simulink model "unrolling_1"  (R2015b)
settings: Solver=FixedStepDiscrete  SolverMode=SingleTasking  StartTime=0.0  StopTime=10.0  RelTol=1e-3
undefined symbols (not defined in the file or in its folder): a, b
libraries: shlslibv1 x4645
(part 1 of 18)
settings Model: synDspstartup=OK  Creator=hchempat  LastModifiedBy=pjampani
settings DataIOCC: SaveOutput=off  SignalLogging=off  SaveTime=off
settings OptimizationCC: DefaultParameterBehavior=Inlined
settings DebuggingCC: AlgebraicLoopMsg=error  InheritedTsInSrcMsg=none

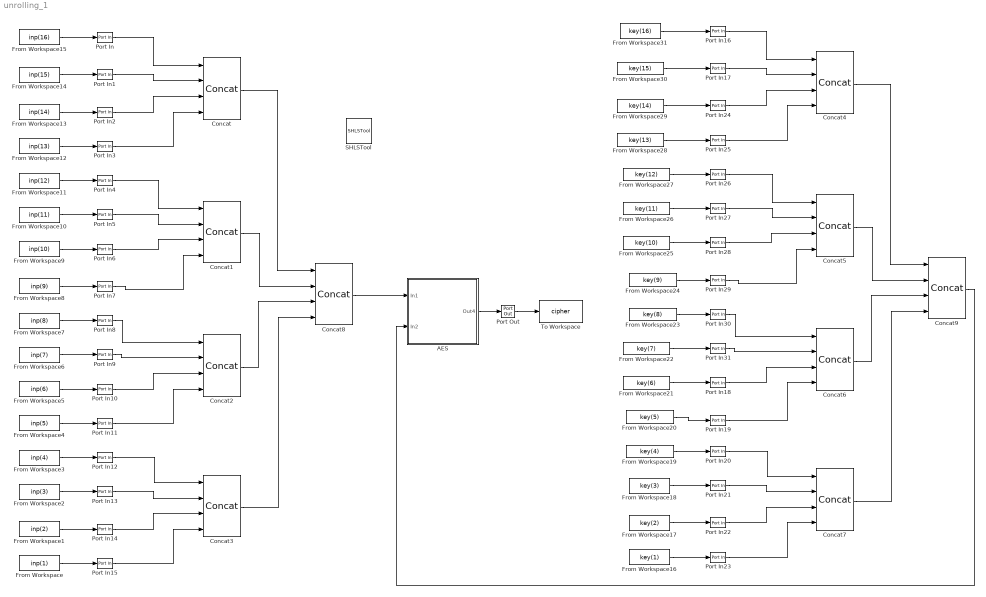
== system unrolling_1 ==
  "AES " : Subsystem
  Concat{,1..9} (10 alike) : shlslibv1/Signal Operations/Concat  syn_in_nb=4  syn_out_f=Automatic  syn_out_wl=16  syn_out_fl=8  syn_out_dt=signed  syn_en_se=off  synBlockType=primitive  synLatency=0  synBlockId=8
  From Workspace : FromWorkspace  VariableName=inp(1)
  From Workspace1 : FromWorkspace  VariableName=inp(2)
  From Workspace10 : FromWorkspace  VariableName=inp(11)
  From Workspace11 : FromWorkspace  VariableName=inp(12)
  From Workspace12 : FromWorkspace  VariableName=inp(13)
  From Workspace13 : FromWorkspace  VariableName=inp(14)
  From Workspace14 : FromWorkspace  VariableName=inp(15)
  From Workspace15 : FromWorkspace  VariableName=inp(16)
  From Workspace16 : FromWorkspace  VariableName=key(1)
  From Workspace17 : FromWorkspace  VariableName=key(2)
  From Workspace18 : FromWorkspace  VariableName=key(3)
  From Workspace19 : FromWorkspace  VariableName=key(4)
  From Workspace2 : FromWorkspace  VariableName=inp(3)
  From Workspace20 : FromWorkspace  VariableName=key(5)
  From Workspace21 : FromWorkspace  VariableName=key(6)
  From Workspace22 : FromWorkspace  VariableName=key(7)
  From Workspace23 : FromWorkspace  VariableName=key(8)
  From Workspace24 : FromWorkspace  VariableName=key(9)
  From Workspace25 : FromWorkspace  VariableName=key(10)
  From Workspace26 : FromWorkspace  VariableName=key(11)
  From Workspace27 : FromWorkspace  VariableName=key(12)
  From Workspace28 : FromWorkspace  VariableName=key(13)
  From Workspace29 : FromWorkspace  VariableName=key(14)
  From Workspace3 : FromWorkspace  VariableName=inp(4)
  From Workspace30 : FromWorkspace  VariableName=key(15)
  From Workspace31 : FromWorkspace  VariableName=key(16)
  From Workspace4 : FromWorkspace  VariableName=inp(5)
  From Workspace5 : FromWorkspace  VariableName=inp(6)
  From Workspace6 : FromWorkspace  VariableName=inp(7)
  From Workspace7 : FromWorkspace  VariableName=inp(8)
  From Workspace8 : FromWorkspace  VariableName=inp(9)
  From Workspace9 : FromWorkspace  VariableName=inp(10)
  Port In{,1..31} (32 alike) : shlslibv1/Ports & Subsystems/Port In  syn_out_wl=8  syn_out_fl=0  syn_out_dt=unsigned  syn_out_st=ts  syn_capture=on  syn_register=on  syn_out_sat=off  syn_out_rnd=on  synBlockType=port  synLatency=1  synBlockId=0
  Port Out : shlslibv1/Ports & Subsystems/Port Out  syn_capture=on  syn_register=on  synBlockType=port  synLatency=1  synBlockId=1
  SHLSTool : shlslibv1/SHLSTool  synBlockType=tool  syn_dsp_mode=FPGA
  To Workspace : ToWorkspace  VariableName=cipher  SaveFormat=Structure With Time  SampleTime=-1
  wires:
  From Workspace15/1 -> Port In/1
  From Workspace14/1 -> Port In1/1
  From Workspace12/1 -> Port In3/1
  From Workspace13/1 -> Port In2/1
  From Workspace11/1 -> Port In4/1
  From Workspace10/1 -> Port In5/1
  From Workspace9/1 -> Port In6/1
  From Workspace8/1 -> Port In7/1
  From Workspace7/1 -> Port In8/1
  From Workspace6/1 -> Port In9/1
  From Workspace5/1 -> Port In10/1
  From Workspace4/1 -> Port In11/1
  From Workspace3/1 -> Port In12/1
  From Workspace2/1 -> Port In13/1
  From Workspace1/1 -> Port In14/1
  From Workspace/1 -> Port In15/1
  Port In2/1 -> Concat/3
  Port In1/1 -> Concat/2
  Port In/1 -> Concat/1
  Port In3/1 -> Concat/4
  Port In6/1 -> Concat1/3
  Port In5/1 -> Concat1/2
  Port In4/1 -> Concat1/1
  Port In7/1 -> Concat1/4
  Port In10/1 -> Concat2/3
  Port In9/1 -> Concat2/2
  Port In8/1 -> Concat2/1
  Port In11/1 -> Concat2/4
  Port In14/1 -> Concat3/3
  Port In13/1 -> Concat3/2
  Port In15/1 -> Concat3/4
  Port In12/1 -> Concat3/1
  From Workspace22/1 -> Port In31/1
  From Workspace21/1 -> Port In18/1
  From Workspace20/1 -> Port In19/1
  From Workspace18/1 -> Port In21/1
  From Workspace17/1 -> Port In22/1
  From Workspace16/1 -> Port In23/1
  Port In24/1 -> Concat4/3
  Port In17/1 -> Concat4/2
  Port In16/1 -> Concat4/1
  Port In25/1 -> Concat4/4
  Port In28/1 -> Concat5/3
  Port In27/1 -> Concat5/2
  Port In26/1 -> Concat5/1
  Port In29/1 -> Concat5/4
  Port In18/1 -> Concat6/3
  Port In31/1 -> Concat6/2
  Port In30/1 -> Concat6/1
  Port In19/1 -> Concat6/4
  Port In22/1 -> Concat7/3
  Port In21/1 -> Concat7/2
  Port In23/1 -> Concat7/4
  Port In20/1 -> Concat7/1
  Concat/1 -> Concat8/1
  Concat1/1 -> Concat8/2
  Concat2/1 -> Concat8/3
  Concat3/1 -> Concat8/4
  Concat4/1 -> Concat9/1
  Concat5/1 -> Concat9/2
  Concat6/1 -> Concat9/3
  Concat7/1 -> Concat9/4
  Port Out/1 -> To Workspace/1
  Concat8/1 -> "AES "/1(In1)
  Concat9/1 -> "AES "/2(In2)
  "AES "/1(Out4) -> Port Out/1
  From Workspace19/1 -> Port In20/1
  From Workspace23/1 -> Port In30/1
  From Workspace24/1 -> Port In29/1
  From Workspace25/1 -> Port In28/1
  From Workspace27/1 -> Port In26/1
  From Workspace28/1 -> Port In25/1
  From Workspace29/1 -> Port In24/1
  From Workspace30/1 -> Port In17/1
  From Workspace31/1 -> Port In16/1
  From Workspace26/1 -> Port In27/1

== system unrolling_1/AES  ==
  In1 : Inport
  In2 : Inport  Port=2
  Concat : shlslibv1/Signal Operations/Concat  syn_in_nb=4  syn_out_f=Automatic  syn_out_wl=16  syn_out_fl=8  syn_out_dt=signed  syn_en_se=off  synBlockType=primitive  synLatency=0  synBlockId=8
  Subsystem : Subsystem
  Subsystem1 : Subsystem
  Subsystem10 : Subsystem
  Subsystem2 : Subsystem
  Subsystem3 : Subsystem
  Subsystem4 : Subsystem
  Subsystem5 : Subsystem
  Subsystem6 : Subsystem
  Subsystem7 : Subsystem
  Subsystem8 : Subsystem
  Subsystem9 : Subsystem
  Out4 : Outport
  wires:
  Subsystem/1(Out1) -> Subsystem1/1(In1)
  Subsystem/2(Out2) -> Subsystem1/2(In2)
  Subsystem/3(Out3) -> Subsystem1/3(In3)
  Subsystem/4(Out4) -> Subsystem1/4(In4)
  Subsystem1/1(Out1) -> Subsystem2/1(In1)
  Subsystem1/2(Out2) -> Subsystem2/2(In2)
  Subsystem1/3(Out3) -> Subsystem2/3(In3)
  Subsystem1/4(Out4) -> Subsystem2/4(In4)
  Subsystem1/5(Out5) -> Subsystem2/5(In5)
  Subsystem2/1(Out1) -> Subsystem3/1(In1)
  Subsystem2/2(Out2) -> Subsystem3/2(In2)
  Subsystem2/3(Out3) -> Subsystem3/3(In3)
  Subsystem2/4(Out4) -> Subsystem3/4(In4)
  Subsystem2/5(Out5) -> Subsystem3/5(In5)
  Subsystem3/1(Out1) -> Subsystem4/1(In1)
  Subsystem3/2(Out2) -> Subsystem4/2(In2)
  Subsystem3/3(Out3) -> Subsystem4/3(In3)
  Subsystem3/4(Out4) -> Subsystem4/4(In4)
  Subsystem3/5(Out5) -> Subsystem4/5(In5)
  Subsystem4/1(Out1) -> Subsystem5/1(In1)
  Subsystem4/2(Out2) -> Subsystem5/2(In2)
  Subsystem4/3(Out3) -> Subsystem5/3(In3)
  Subsystem4/4(Out4) -> Subsystem5/4(In4)
  Subsystem4/5(Out5) -> Subsystem5/5(In5)
  Subsystem5/1(Out1) -> Subsystem6/1(In1)
  Subsystem5/2(Out2) -> Subsystem6/2(In2)
  Subsystem5/3(Out3) -> Subsystem6/3(In3)
  Subsystem5/4(Out4) -> Subsystem6/4(In4)
  Subsystem5/5(Out5) -> Subsystem6/5(In5)
  Subsystem6/1(Out1) -> Subsystem7/1(In1)
  Subsystem6/2(Out2) -> Subsystem7/2(In2)
  Subsystem6/3(Out3) -> Subsystem7/3(In3)
  Subsystem6/4(Out4) -> Subsystem7/4(In4)
  Subsystem6/5(Out5) -> Subsystem7/5(In5)
  Subsystem7/5(Out5) -> Subsystem8/5(In5)
  Subsystem7/4(Out4) -> Subsystem8/4(In4)
  Subsystem7/3(Out3) -> Subsystem8/3(In3)
  Subsystem7/2(Out2) -> Subsystem8/2(In2)
  Subsystem8/1(Out1) -> Subsystem9/1(In1)
  Subsystem8/2(Out2) -> Subsystem9/2(In2)
  Subsystem8/5(Out5) -> Subsystem9/5(In5)
  Subsystem8/4(Out4) -> Subsystem9/4(In4)
  Subsystem8/3(Out3) -> Subsystem9/3(In3)
  Subsystem9/1(Out1) -> Subsystem10/1(In1)
  Subsystem9/2(Out2) -> Subsystem10/2(In2)
  Subsystem9/3(Out3) -> Subsystem10/3(In3)
  Subsystem9/4(Out4) -> Subsystem10/4(In4)
  Subsystem9/5(Out5) -> Subsystem10/5(In5)
  Subsystem10/4(Out4) -> Concat/4
  Subsystem10/3(Out3) -> Concat/3
  Subsystem10/2(Out2) -> Concat/2
  Subsystem10/1(Out1) -> Concat/1
  In2/1 -> Subsystem1/5(In5), Subsystem/2(In2)
  In1/1 -> Subsystem/1(In1)
  Concat/1 -> Out4/1
  Subsystem7/1(Out1) -> Subsystem8/1(In1)

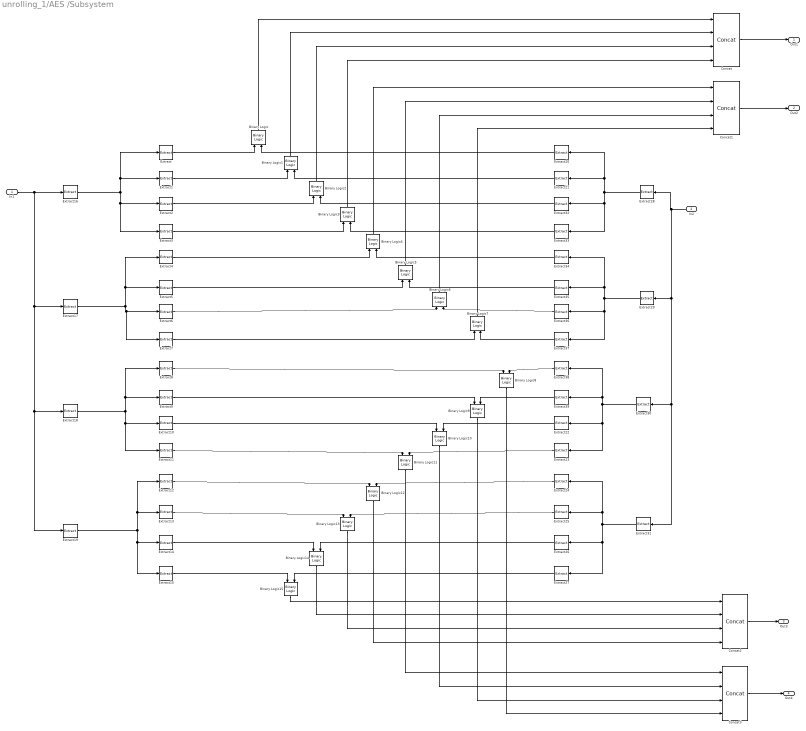
== system unrolling_1/AES /Subsystem ==
  In1 : Inport
  In2 : Inport  Port=2
  Binary Logic{,1..15} (16 alike) : shlslibv1/Math Functions/Binary Logic  syn_binlog_exp=a^b  synBlockType=primitive  synLatency=0  synBlockId=13
  Concat{,1..3} (4 alike) : shlslibv1/Signal Operations/Concat  syn_in_nb=4  syn_out_f=Automatic  syn_out_wl=16  syn_out_fl=8  syn_out_dt=signed  syn_en_se=off  synBlockType=primitive  synLatency=0  synBlockId=8
  Extract{,4,8,12,20,24,34,38} (8 alike) : shlslibv1/Signal Operations/Extract  syn_extract_vec=[24:31]  synBlockType=primitive  synLatency=0  synBlockId=17
  Extract{1,5,9,13,21,25,35,39} (8 alike) : shlslibv1/Signal Operations/Extract  syn_extract_vec=[16:23]  synBlockType=primitive  synLatency=0  synBlockId=17
  Extract{2,6,10,14,22,26,32,36} (8 alike) : shlslibv1/Signal Operations/Extract  syn_extract_vec=[8:15]  synBlockType=primitive  synLatency=0  synBlockId=17
  Extract{3,7,11,15,23,27,33,37} (8 alike) : shlslibv1/Signal Operations/Extract  syn_extract_vec=[0:7]  synBlockType=primitive  synLatency=0  synBlockId=17
  Extract16 : shlslibv1/Signal Operations/Extract  syn_extract_vec=[96:127]  synBlockType=primitive  synLatency=0  synBlockId=17
  Extract17 : shlslibv1/Signal Operations/Extract  syn_extract_vec=[64:95]  synBlockType=primitive  synLatency=0  synBlockId=17
  Extract18 : shlslibv1/Signal Operations/Extract  syn_extract_vec=[32:63]  synBlockType=primitive  synLatency=0  synBlockId=17
  Extract19 : shlslibv1/Signal Operations/Extract  syn_extract_vec=[0:31]  synBlockType=primitive  synLatency=0  synBlockId=17
  Extract28 : shlslibv1/Signal Operations/Extract  syn_extract_vec=[96:127]  synBlockType=primitive  synLatency=0  synBlockId=17
  Extract29 : shlslibv1/Signal Operations/Extract  syn_extract_vec=[64:95]  synBlockType=primitive  synLatency=0  synBlockId=17
  Extract30 : shlslibv1/Signal Operations/Extract  syn_extract_vec=[32:63]  synBlockType=primitive  synLatency=0  synBlockId=17
  Extract31 : shlslibv1/Signal Operations/Extract  syn_extract_vec=[0:31]  synBlockType=primitive  synLatency=0  synBlockId=17
  Out1 : Outport
  Out2 : Outport  Port=2
  Out3 : Outport  Port=3
  Out4 : Outport  Port=4
  wires:
  Extract16/1 -> Extract/1, Extract1/1, Extract2/1, Extract3/1
  Extract17/1 -> Extract6/1, Extract7/1, Extract4/1, Extract5/1
  Extract18/1 -> Extract9/1, Extract8/1, Extract10/1, Extract11/1
  Extract19/1 -> Extract12/1, Extract13/1, Extract15/1, Extract14/1
  In1/1 -> Extract19/1, Extract18/1, Extract17/1, Extract16/1
  In2/1 -> Extract31/1, Extract30/1, Extract29/1, Extract28/1
  Extract28/1 -> Extract21/1, Extract20/1, Extract33/1, Extract32/1
  Extract29/1 -> Extract35/1, Extract34/1, Extract36/1, Extract37/1
  Extract30/1 -> Extract23/1, Extract22/1, Extract38/1, Extract39/1
  Extract31/1 -> Extract24/1, Extract25/1, Extract27/1, Extract26/1
  Extract/1 -> Binary Logic/1
  Extract20/1 -> Binary Logic/2
  Extract1/1 -> Binary Logic1/1
  Extract21/1 -> Binary Logic1/2
  Extract2/1 -> Binary Logic2/1
  Extract32/1 -> Binary Logic2/2
  Extract3/1 -> Binary Logic3/1
  Extract33/1 -> Binary Logic3/2
  Extract4/1 -> Binary Logic4/1
  Extract34/1 -> Binary Logic4/2
  Extract5/1 -> Binary Logic5/1
  Extract35/1 -> Binary Logic5/2
  Extract6/1 -> Binary Logic6/1
  Extract36/1 -> Binary Logic6/2
  Extract7/1 -> Binary Logic7/1
  Extract37/1 -> Binary Logic7/2
  Extract8/1 -> Binary Logic8/1
  Extract38/1 -> Binary Logic8/2
  Extract9/1 -> Binary Logic9/1
  Extract39/1 -> Binary Logic9/2
  Extract22/1 -> Binary Logic10/2
  Extract10/1 -> Binary Logic10/1
  Extract23/1 -> Binary Logic11/2
  Extract11/1 -> Binary Logic11/1
  Extract12/1 -> Binary Logic12/1
  Extract24/1 -> Binary Logic12/2
  Extract13/1 -> Binary Logic13/1
  Extract25/1 -> Binary Logic13/2
  Extract14/1 -> Binary Logic14/1
  Extract26/1 -> Binary Logic14/2
  Extract15/1 -> Binary Logic15/1
  Extract27/1 -> Binary Logic15/2
  Binary Logic7/1 -> Concat1/4
  Binary Logic6/1 -> Concat1/3
  Binary Logic5/1 -> Concat1/2
  Binary Logic4/1 -> Concat1/1
  Binary Logic3/1 -> Concat/4
  Binary Logic2/1 -> Concat/3
  Binary Logic1/1 -> Concat/2
  Binary Logic/1 -> Concat/1
  Binary Logic15/1 -> Concat2/1
  Binary Logic14/1 -> Concat2/2
  Binary Logic13/1 -> Concat2/3
  Binary Logic12/1 -> Concat2/4
  Binary Logic11/1 -> Concat3/1
  Binary Logic10/1 -> Concat3/2
  Binary Logic9/1 -> Concat3/3
  Binary Logic8/1 -> Concat3/4
  Concat/1 -> Out1/1
  Concat1/1 -> Out2/1
  Concat2/1 -> Out3/1
  Concat3/1 -> Out4/1

== system unrolling_1/AES /Subsystem1 ==
  In1 : Inport
  In2 : Inport  Port=2
  In3 : Inport  Port=3
  In4 : Inport  Port=4
  In5 : Inport  Port=5
  ADD ROUND KEY : Subsystem
  KEYEXPANSION : Subsystem
  SB_rs_MIX_COLUMN : Subsystem
  Out1 : Outport
  Out2 : Outport  Port=2
  Out3 : Outport  Port=3
  Out4 : Outport  Port=4
  Out5 : Outport  Port=5
  wires:
  SB_rs_MIX_COLUMN/1(Out1) -> ADD ROUND KEY/1(In1)
  KEYEXPANSION/1(Out1) -> Out5/1, ADD ROUND KEY/2(In2)
  In1/1 -> SB_rs_MIX_COLUMN/1(In1)
  In2/1 -> SB_rs_MIX_COLUMN/2(In2)
  In3/1 -> SB_rs_MIX_COLUMN/3(In3)
  In4/1 -> SB_rs_MIX_COLUMN/4(In4)
  In5/1 -> KEYEXPANSION/1(In1)
  ADD ROUND KEY/1(Out1) -> Out1/1
  ADD ROUND KEY/2(Out2) -> Out2/1
  ADD ROUND KEY/3(Out3) -> Out3/1
  ADD ROUND KEY/4(Out4) -> Out4/1

== system unrolling_1/AES /Subsystem10 ==
  In1 : Inport
  In2 : Inport  Port=2
  In3 : Inport  Port=3
  In4 : Inport  Port=4
  In5 : Inport  Port=5
  ADD ROUND KEY : Subsystem
  KEYEXPANSION : Subsystem
  SB_rs_MIX_COLUMN : Subsystem
  Out1 : Outport
  Out2 : Outport  Port=2
  Out3 : Outport  Port=3
  Out4 : Outport  Port=4
  wires:
  SB_rs_MIX_COLUMN/1(Out1) -> ADD ROUND KEY/1(In1)
  KEYEXPANSION/1(Out1) -> ADD ROUND KEY/2(In2)
  In1/1 -> SB_rs_MIX_COLUMN/1(In1)
  In2/1 -> SB_rs_MIX_COLUMN/2(In2)
  In3/1 -> SB_rs_MIX_COLUMN/3(In3)
  In4/1 -> SB_rs_MIX_COLUMN/4(In4)
  In5/1 -> KEYEXPANSION/1(In1)
  ADD ROUND KEY/1(Out1) -> Out1/1
  ADD ROUND KEY/2(Out2) -> Out2/1
  ADD ROUND KEY/3(Out3) -> Out3/1
  ADD ROUND KEY/4(Out4) -> Out4/1

== system unrolling_1/AES /Subsystem2 ==
  In1 : Inport
  In2 : Inport  Port=2
  In3 : Inport  Port=3
  In4 : Inport  Port=4
  In5 : Inport  Port=5
  ADD ROUND KEY : Subsystem
  KEYEXPANSION : Subsystem
  SB_rs_MIX_COLUMN : Subsystem
  Out1 : Outport
  Out2 : Outport  Port=2
  Out3 : Outport  Port=3
  Out4 : Outport  Port=4
  Out5 : Outport  Port=5
  wires:
  SB_rs_MIX_COLUMN/1(Out1) -> ADD ROUND KEY/1(In1)
  KEYEXPANSION/1(Out1) -> Out5/1, ADD ROUND KEY/2(In2)
  In1/1 -> SB_rs_MIX_COLUMN/1(In1)
  In2/1 -> SB_rs_MIX_COLUMN/2(In2)
  In3/1 -> SB_rs_MIX_COLUMN/3(In3)
  In4/1 -> SB_rs_MIX_COLUMN/4(In4)
  In5/1 -> KEYEXPANSION/1(In1)
  ADD ROUND KEY/1(Out1) -> Out1/1
  ADD ROUND KEY/2(Out2) -> Out2/1
  ADD ROUND KEY/3(Out3) -> Out3/1
  ADD ROUND KEY/4(Out4) -> Out4/1

== system unrolling_1/AES /Subsystem3 ==
  In1 : Inport
  In2 : Inport  Port=2
  In3 : Inport  Port=3
  In4 : Inport  Port=4
  In5 : Inport  Port=5
  ADD ROUND KEY : Subsystem
  KEYEXPANSION : Subsystem
  SB_rs_MIX_COLUMN : Subsystem
  Out1 : Outport
  Out2 : Outport  Port=2
  Out3 : Outport  Port=3
  Out4 : Outport  Port=4
  Out5 : Outport  Port=5
  wires:
  SB_rs_MIX_COLUMN/1(Out1) -> ADD ROUND KEY/1(In1)
  KEYEXPANSION/1(Out1) -> Out5/1, ADD ROUND KEY/2(In2)
  In1/1 -> SB_rs_MIX_COLUMN/1(In1)
  In2/1 -> SB_rs_MIX_COLUMN/2(In2)
  In3/1 -> SB_rs_MIX_COLUMN/3(In3)
  In4/1 -> SB_rs_MIX_COLUMN/4(In4)
  In5/1 -> KEYEXPANSION/1(In1)
  ADD ROUND KEY/1(Out1) -> Out1/1
  ADD ROUND KEY/2(Out2) -> Out2/1
  ADD ROUND KEY/3(Out3) -> Out3/1
  ADD ROUND KEY/4(Out4) -> Out4/1

== system unrolling_1/AES /Subsystem4 ==
  In1 : Inport
  In2 : Inport  Port=2
  In3 : Inport  Port=3
  In4 : Inport  Port=4
  In5 : Inport  Port=5
  ADD ROUND KEY : Subsystem
  KEYEXPANSION : Subsystem
  SB_rs_MIX_COLUMN : Subsystem
  Out1 : Outport
  Out2 : Outport  Port=2
  Out3 : Outport  Port=3
  Out4 : Outport  Port=4
  Out5 : Outport  Port=5
  wires:
  SB_rs_MIX_COLUMN/1(Out1) -> ADD ROUND KEY/1(In1)
  KEYEXPANSION/1(Out1) -> Out5/1, ADD ROUND KEY/2(In2)
  In1/1 -> SB_rs_MIX_COLUMN/1(In1)
  In2/1 -> SB_rs_MIX_COLUMN/2(In2)
  In3/1 -> SB_rs_MIX_COLUMN/3(In3)
  In4/1 -> SB_rs_MIX_COLUMN/4(In4)
  In5/1 -> KEYEXPANSION/1(In1)
  ADD ROUND KEY/1(Out1) -> Out1/1
  ADD ROUND KEY/2(Out2) -> Out2/1
  ADD ROUND KEY/3(Out3) -> Out3/1
  ADD ROUND KEY/4(Out4) -> Out4/1

== system unrolling_1/AES /Subsystem5 ==
  In1 : Inport
  In2 : Inport  Port=2
  In3 : Inport  Port=3
  In4 : Inport  Port=4
  In5 : Inport  Port=5
  ADD ROUND KEY : Subsystem
  KEYEXPANSION : Subsystem
  SB_rs_MIX_COLUMN : Subsystem
  Out1 : Outport
  Out2 : Outport  Port=2
  Out3 : Outport  Port=3
  Out4 : Outport  Port=4
  Out5 : Outport  Port=5
  wires:
  SB_rs_MIX_COLUMN/1(Out1) -> ADD ROUND KEY/1(In1)
  KEYEXPANSION/1(Out1) -> Out5/1, ADD ROUND KEY/2(In2)
  In1/1 -> SB_rs_MIX_COLUMN/1(In1)
  In2/1 -> SB_rs_MIX_COLUMN/2(In2)
  In3/1 -> SB_rs_MIX_COLUMN/3(In3)
  In4/1 -> SB_rs_MIX_COLUMN/4(In4)
  In5/1 -> KEYEXPANSION/1(In1)
  ADD ROUND KEY/1(Out1) -> Out1/1
  ADD ROUND KEY/2(Out2) -> Out2/1
  ADD ROUND KEY/3(Out3) -> Out3/1
  ADD ROUND KEY/4(Out4) -> Out4/1

== system unrolling_1/AES /Subsystem6 ==
  In1 : Inport
  In2 : Inport  Port=2
  In3 : Inport  Port=3
  In4 : Inport  Port=4
  In5 : Inport  Port=5
  ADD ROUND KEY : Subsystem
  KEYEXPANSION : Subsystem
  SB_rs_MIX_COLUMN : Subsystem
  Out1 : Outport
  Out2 : Outport  Port=2
  Out3 : Outport  Port=3
  Out4 : Outport  Port=4
  Out5 : Outport  Port=5
  wires:
  SB_rs_MIX_COLUMN/1(Out1) -> ADD ROUND KEY/1(In1)
  KEYEXPANSION/1(Out1) -> Out5/1, ADD ROUND KEY/2(In2)
  In1/1 -> SB_rs_MIX_COLUMN/1(In1)
  In2/1 -> SB_rs_MIX_COLUMN/2(In2)
  In3/1 -> SB_rs_MIX_COLUMN/3(In3)
  In4/1 -> SB_rs_MIX_COLUMN/4(In4)
  In5/1 -> KEYEXPANSION/1(In1)
  ADD ROUND KEY/1(Out1) -> Out1/1
  ADD ROUND KEY/2(Out2) -> Out2/1
  ADD ROUND KEY/3(Out3) -> Out3/1
  ADD ROUND KEY/4(Out4) -> Out4/1

== system unrolling_1/AES /Subsystem7 ==
  In1 : Inport
  In2 : Inport  Port=2
  In3 : Inport  Port=3
  In4 : Inport  Port=4
  In5 : Inport  Port=5
  ADD ROUND KEY : Subsystem
  KEYEXPANSION : Subsystem
  SB_rs_MIX_COLUMN : Subsystem
  Out1 : Outport
  Out2 : Outport  Port=2
  Out3 : Outport  Port=3
  Out4 : Outport  Port=4
  Out5 : Outport  Port=5
  wires:
  SB_rs_MIX_COLUMN/1(Out1) -> ADD ROUND KEY/1(In1)
  KEYEXPANSION/1(Out1) -> Out5/1, ADD ROUND KEY/2(In2)
  In1/1 -> SB_rs_MIX_COLUMN/1(In1)
  In2/1 -> SB_rs_MIX_COLUMN/2(In2)
  In3/1 -> SB_rs_MIX_COLUMN/3(In3)
  In4/1 -> SB_rs_MIX_COLUMN/4(In4)
  In5/1 -> KEYEXPANSION/1(In1)
  ADD ROUND KEY/1(Out1) -> Out1/1
  ADD ROUND KEY/2(Out2) -> Out2/1
  ADD ROUND KEY/3(Out3) -> Out3/1
  ADD ROUND KEY/4(Out4) -> Out4/1

== system unrolling_1/AES /Subsystem8 ==
  In1 : Inport
  In2 : Inport  Port=2
  In3 : Inport  Port=3
  In4 : Inport  Port=4
  In5 : Inport  Port=5
  ADD ROUND KEY : Subsystem
  KEYEXPANSION : Subsystem
  SB_rs_MIX_COLUMN : Subsystem
  Out1 : Outport
  Out2 : Outport  Port=2
  Out3 : Outport  Port=3
  Out4 : Outport  Port=4
  Out5 : Outport  Port=5
  wires:
  SB_rs_MIX_COLUMN/1(Out1) -> ADD ROUND KEY/1(In1)
  KEYEXPANSION/1(Out1) -> Out5/1, ADD ROUND KEY/2(In2)
  In1/1 -> SB_rs_MIX_COLUMN/1(In1)
  In2/1 -> SB_rs_MIX_COLUMN/2(In2)
  In3/1 -> SB_rs_MIX_COLUMN/3(In3)
  In4/1 -> SB_rs_MIX_COLUMN/4(In4)
  In5/1 -> KEYEXPANSION/1(In1)
  ADD ROUND KEY/1(Out1) -> Out1/1
  ADD ROUND KEY/2(Out2) -> Out2/1
  ADD ROUND KEY/3(Out3) -> Out3/1
  ADD ROUND KEY/4(Out4) -> Out4/1

== system unrolling_1/AES /Subsystem9 ==
  In1 : Inport
  In2 : Inport  Port=2
  In3 : Inport  Port=3
  In4 : Inport  Port=4
  In5 : Inport  Port=5
  ADD ROUND KEY : Subsystem
  KEYEXPANSION : Subsystem
  SB_rs_MIX_COLUMN : Subsystem
  Out1 : Outport
  Out2 : Outport  Port=2
  Out3 : Outport  Port=3
  Out4 : Outport  Port=4
  Out5 : Outport  Port=5
  wires:
  SB_rs_MIX_COLUMN/1(Out1) -> ADD ROUND KEY/1(In1)
  KEYEXPANSION/1(Out1) -> Out5/1, ADD ROUND KEY/2(In2)
  In1/1 -> SB_rs_MIX_COLUMN/1(In1)
  In2/1 -> SB_rs_MIX_COLUMN/2(In2)
  In3/1 -> SB_rs_MIX_COLUMN/3(In3)
  In4/1 -> SB_rs_MIX_COLUMN/4(In4)
  In5/1 -> KEYEXPANSION/1(In1)
  ADD ROUND KEY/1(Out1) -> Out1/1
  ADD ROUND KEY/2(Out2) -> Out2/1
  ADD ROUND KEY/3(Out3) -> Out3/1
  ADD ROUND KEY/4(Out4) -> Out4/1

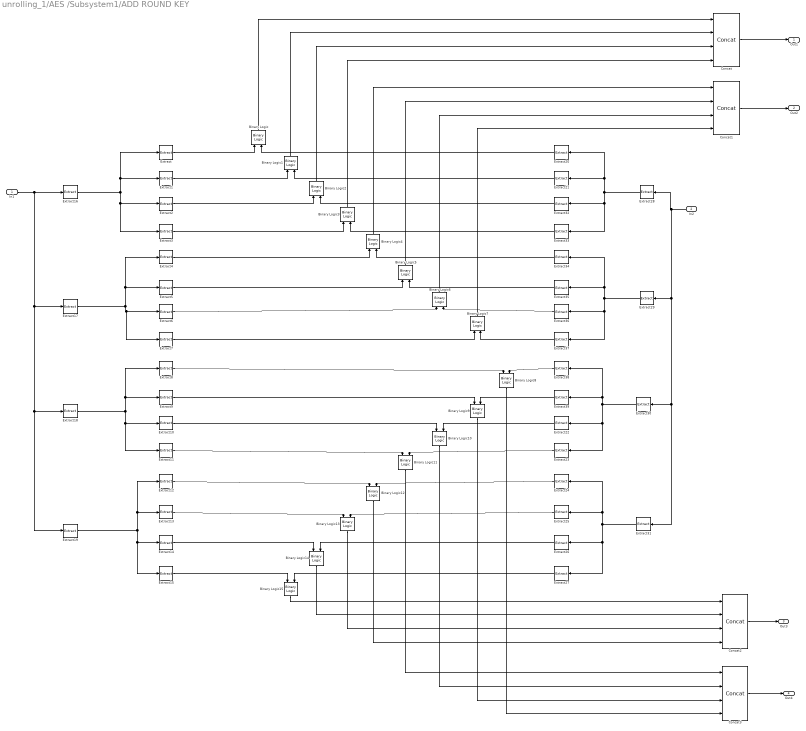
== system unrolling_1/AES /Subsystem1/ADD ROUND KEY ==
  In1 : Inport
  In2 : Inport  Port=2
  Binary Logic{,1..15} (16 alike) : shlslibv1/Math Functions/Binary Logic  syn_binlog_exp=a^b  synBlockType=primitive  synLatency=0  synBlockId=13
  Concat{,1..3} (4 alike) : shlslibv1/Signal Operations/Concat  syn_in_nb=4  syn_out_f=Automatic  syn_out_wl=16  syn_out_fl=8  syn_out_dt=signed  syn_en_se=off  synBlockType=primitive  synLatency=0  synBlockId=8
  Extract{,4,8,12,20,24,34,38} (8 alike) : shlslibv1/Signal Operations/Extract  syn_extract_vec=[24:31]  synBlockType=primitive  synLatency=0  synBlockId=17
  Extract{1,5,9,13,21,25,35,39} (8 alike) : shlslibv1/Signal Operations/Extract  syn_extract_vec=[16:23]  synBlockType=primitive  synLatency=0  synBlockId=17
  Extract{2,6,10,14,22,26,32,36} (8 alike) : shlslibv1/Signal Operations/Extract  syn_extract_vec=[8:15]  synBlockType=primitive  synLatency=0  synBlockId=17
  Extract{3,7,11,15,23,27,33,37} (8 alike) : shlslibv1/Signal Operations/Extract  syn_extract_vec=[0:7]  synBlockType=primitive  synLatency=0  synBlockId=17
  Extract16 : shlslibv1/Signal Operations/Extract  syn_extract_vec=[96:127]  synBlockType=primitive  synLatency=0  synBlockId=17
  Extract17 : shlslibv1/Signal Operations/Extract  syn_extract_vec=[64:95]  synBlockType=primitive  synLatency=0  synBlockId=17
  Extract18 : shlslibv1/Signal Operations/Extract  syn_extract_vec=[32:63]  synBlockType=primitive  synLatency=0  synBlockId=17
  Extract19 : shlslibv1/Signal Operations/Extract  syn_extract_vec=[0:31]  synBlockType=primitive  synLatency=0  synBlockId=17
  Extract28 : shlslibv1/Signal Operations/Extract  syn_extract_vec=[96:127]  synBlockType=primitive  synLatency=0  synBlockId=17
  Extract29 : shlslibv1/Signal Operations/Extract  syn_extract_vec=[64:95]  synBlockType=primitive  synLatency=0  synBlockId=17
  Extract30 : shlslibv1/Signal Operations/Extract  syn_extract_vec=[32:63]  synBlockType=primitive  synLatency=0  synBlockId=17
  Extract31 : shlslibv1/Signal Operations/Extract  syn_extract_vec=[0:31]  synBlockType=primitive  synLatency=0  synBlockId=17
  Out1 : Outport
  Out2 : Outport  Port=2
  Out3 : Outport  Port=3
  Out4 : Outport  Port=4
  wires:
  Extract16/1 -> Extract/1, Extract1/1, Extract2/1, Extract3/1
  Extract17/1 -> Extract6/1, Extract7/1, Extract4/1, Extract5/1
  Extract18/1 -> Extract9/1, Extract8/1, Extract10/1, Extract11/1
  Extract19/1 -> Extract12/1, Extract13/1, Extract15/1, Extract14/1
  In1/1 -> Extract19/1, Extract18/1, Extract17/1, Extract16/1
  In2/1 -> Extract31/1, Extract30/1, Extract29/1, Extract28/1
  Extract28/1 -> Extract21/1, Extract20/1, Extract33/1, Extract32/1
  Extract29/1 -> Extract35/1, Extract34/1, Extract36/1, Extract37/1
  Extract30/1 -> Extract23/1, Extract22/1, Extract38/1, Extract39/1
  Extract31/1 -> Extract24/1, Extract25/1, Extract27/1, Extract26/1
  Extract/1 -> Binary Logic/1
  Extract20/1 -> Binary Logic/2
  Extract1/1 -> Binary Logic1/1
  Extract21/1 -> Binary Logic1/2
  Extract2/1 -> Binary Logic2/1
  Extract32/1 -> Binary Logic2/2
  Extract3/1 -> Binary Logic3/1
  Extract33/1 -> Binary Logic3/2
  Extract4/1 -> Binary Logic4/1
  Extract34/1 -> Binary Logic4/2
  Extract5/1 -> Binary Logic5/1
  Extract35/1 -> Binary Logic5/2
  Extract6/1 -> Binary Logic6/1
  Extract36/1 -> Binary Logic6/2
  Extract7/1 -> Binary Logic7/1
  Extract37/1 -> Binary Logic7/2
  Extract8/1 -> Binary Logic8/1
  Extract38/1 -> Binary Logic8/2
  Extract9/1 -> Binary Logic9/1
  Extract39/1 -> Binary Logic9/2
  Extract22/1 -> Binary Logic10/2
  Extract10/1 -> Binary Logic10/1
  Extract23/1 -> Binary Logic11/2
  Extract11/1 -> Binary Logic11/1
  Extract12/1 -> Binary Logic12/1
  Extract24/1 -> Binary Logic12/2
  Extract13/1 -> Binary Logic13/1
  Extract25/1 -> Binary Logic13/2
  Extract14/1 -> Binary Logic14/1
  Extract26/1 -> Binary Logic14/2
  Extract15/1 -> Binary Logic15/1
  Extract27/1 -> Binary Logic15/2
  Binary Logic7/1 -> Concat1/4
  Binary Logic6/1 -> Concat1/3
  Binary Logic5/1 -> Concat1/2
  Binary Logic4/1 -> Concat1/1
  Binary Logic3/1 -> Concat/4
  Binary Logic2/1 -> Concat/3
  Binary Logic1/1 -> Concat/2
  Binary Logic/1 -> Concat/1
  Binary Logic15/1 -> Concat2/1
  Binary Logic14/1 -> Concat2/2
  Binary Logic13/1 -> Concat2/3
  Binary Logic12/1 -> Concat2/4
  Binary Logic11/1 -> Concat3/1
  Binary Logic10/1 -> Concat3/2
  Binary Logic9/1 -> Concat3/3
  Binary Logic8/1 -> Concat3/4
  Concat/1 -> Out1/1
  Concat1/1 -> Out2/1
  Concat2/1 -> Out3/1
  Concat3/1 -> Out4/1

== system unrolling_1/AES /Subsystem1/KEYEXPANSION ==
  In1 : Inport
  Binary Logic{,1..19} (20 alike) : shlslibv1/Math Functions/Binary Logic  syn_binlog_exp=a^b  synBlockType=primitive  synLatency=0  synBlockId=13
  Concat{,1..4} (5 alike) : shlslibv1/Signal Operations/Concat  syn_in_nb=4  syn_out_f=Automatic  syn_out_wl=16  syn_out_fl=8  syn_out_dt=signed  syn_en_se=off  synBlockType=primitive  synLatency=0  synBlockId=8
  Constant : shlslibv1/Sources/Constant  syn_cst_val=0  syn_cst_format=Specify  syn_cst_wl=8  syn_cst_fl=0  syn_cst_dt=unsigned  syn_cst_rnd=on  syn_cst_st=-1  synBlockType=primitive  synLatency=0  synBlockId=15
  Constant1 : shlslibv1/Sources/Constant  syn_cst_val=0  syn_cst_format=Specify  syn_cst_wl=8  syn_cst_fl=0  syn_cst_dt=unsigned  syn_cst_rnd=on  syn_cst_st=-1  synBlockType=primitive  synLatency=0  synBlockId=15
  Constant10 : shlslibv1/Sources/Constant  syn_cst_val=64  syn_cst_format=Specify  syn_cst_wl=8  syn_cst_fl=0  syn_cst_dt=unsigned  syn_cst_rnd=on  syn_cst_st=-1  synBlockType=primitive  synLatency=0  synBlockId=15
  Constant11 : shlslibv1/Sources/Constant  syn_cst_val=32  syn_cst_format=Specify  syn_cst_wl=8  syn_cst_fl=0  syn_cst_dt=unsigned  syn_cst_rnd=on  syn_cst_st=-1  synBlockType=primitive  synLatency=0  synBlockId=15
  Constant12 : shlslibv1/Sources/Constant  syn_cst_val=16  syn_cst_format=Specify  syn_cst_wl=8  syn_cst_fl=0  syn_cst_dt=unsigned  syn_cst_rnd=on  syn_cst_st=-1  synBlockType=primitive  synLatency=0  synBlockId=15
  Constant2 : shlslibv1/Sources/Constant  syn_cst_val=0  syn_cst_format=Specify  syn_cst_wl=8  syn_cst_fl=0  syn_cst_dt=unsigned  syn_cst_rnd=on  syn_cst_st=-1  synBlockType=primitive  synLatency=0  synBlockId=15
  Constant4 : shlslibv1/Sources/Constant  syn_cst_val=1  syn_cst_format=Specify  syn_cst_wl=8  syn_cst_fl=0  syn_cst_dt=unsigned  syn_cst_rnd=on  syn_cst_st=-1  synBlockType=primitive  synLatency=0  synBlockId=15
  Constant5 : shlslibv1/Sources/Constant  syn_cst_val=2  syn_cst_format=Specify  syn_cst_wl=8  syn_cst_fl=0  syn_cst_dt=unsigned  syn_cst_rnd=on  syn_cst_st=-1  synBlockType=primitive  synLatency=0  synBlockId=15
  Constant6 : shlslibv1/Sources/Constant  syn_cst_val=4  syn_cst_format=Specify  syn_cst_wl=8  syn_cst_fl=0  syn_cst_dt=unsigned  syn_cst_rnd=on  syn_cst_st=-1  synBlockType=primitive  synLatency=0  synBlockId=15
  Constant7 : shlslibv1/Sources/Constant  syn_cst_val=8  syn_cst_format=Specify  syn_cst_wl=8  syn_cst_fl=0  syn_cst_dt=unsigned  syn_cst_rnd=on  syn_cst_st=-1  synBlockType=primitive  synLatency=0  synBlockId=15
  Constant8 : shlslibv1/Sources/Constant  syn_cst_val=27  syn_cst_format=Specify  syn_cst_wl=8  syn_cst_fl=0  syn_cst_dt=unsigned  syn_cst_rnd=on  syn_cst_st=-1  synBlockType=primitive  synLatency=0  synBlockId=15
  Constant9 : shlslibv1/Sources/Constant  syn_cst_val=128  syn_cst_format=Specify  syn_cst_wl=8  syn_cst_fl=0  syn_cst_dt=unsigned  syn_cst_rnd=on  syn_cst_st=-1  synBlockType=primitive  synLatency=0  synBlockId=15
  Extract1 : shlslibv1/Signal Operations/Extract  syn_extract_vec=[96:127]  synBlockType=primitive  synLatency=0  synBlockId=17
  Extract{6,10,14,18} (4 alike) : shlslibv1/Signal Operations/Extract  syn_extract_vec=[16:23]  synBlockType=primitive  synLatency=0  synBlockId=17
  Extract{7,11,15,19} (4 alike) : shlslibv1/Signal Operations/Extract  syn_extract_vec=[8:15]  synBlockType=primitive  synLatency=0  synBlockId=17
  Extract{8,12,16,20} (4 alike) : shlslibv1/Signal Operations/Extract  syn_extract_vec=[0:7]  synBlockType=primitive  synLatency=0  synBlockId=17
  Extract{5,9,13,17} (4 alike) : shlslibv1/Signal Operations/Extract  syn_extract_vec=[24:31]  synBlockType=primitive  synLatency=0  synBlockId=17
  Extract2 : shlslibv1/Signal Operations/Extract  syn_extract_vec=[64:95]  synBlockType=primitive  synLatency=0  synBlockId=17
  Extract3 : shlslibv1/Signal Operations/Extract  syn_extract_vec=[32:63]  synBlockType=primitive  synLatency=0  synBlockId=17
  Extract4 : shlslibv1/Signal Operations/Extract  syn_extract_vec=[0:31]  synBlockType=primitive  synLatency=0  synBlockId=17
  Mux : shlslibv1/Signal Operations/Mux  syn_in_nb=9  syn_out_f=Full Precision  syn_out_wl=16  syn_out_fl=8  syn_out_dt=signed  syn_en_se=off  synBlockType=primitive  synLatency=0  synBlockId=16
  ROM : shlslibv1/Memories/ROM  syn_rom_vec=[99 124 119 123 242 107 111 197 48 1 103 43 254 215 171 118 202 130 201 125 250 89 71 240 173 212 162 175 156 164 114 192 183 253 147 38 54 63 247 204 52 165 229 241 113 216 49 21 4 199 35 195 24 150 5 154 7 18 128 226 235 39 178 117 9 131 44 26 27 110 90 160 82 59 214 179 41 227 47 132 83 209 0 237 32 252 177 91 106 203 190 57 74 76 88 207 208 239 170 251 67 77 51 133 69 249 2 127 80 60 159 168 81 163 64 143 146 157 56 245 188 182 218 33 16 255 243 210 205 12 19 236 95 151 68 23 196 167 126 61 100 93 25 115 96 129 79 220 34 42 144 136 70 238 184 20 222 94 11 219 224 50 58 10 73 6 36 92 194 211 172 98 145 149 228 121 231 200 55 109 141 213 78 169 108 86 244 234 101 122 174 8 186 120 37 46 28 166 180 198 232 221 116 31 75 189 139 138 112 62 181 102 72 3 246 14 97 53 87 185 134 193 29 158 225 248 152 17 105 217 142 148 155 30 135 233 206 85 40 223 140 161 137 13 191 230 66 104 65 153 45 15 176 84 187 22]  syn_rom_auto_wl=off  syn_out_wl=8  syn_out_fl=0  syn_out_dt=unsigned  syn_out_sat=on  syn_out_rnd=on  syn_en_port=off  synBlockType=primitive  synLatency=1  synBlockId=62  syn_dual_port=on
  ROM1 : shlslibv1/Memories/ROM  syn_rom_vec=[99 124 119 123 242 107 111 197 48 1 103 43 254 215 171 118 202 130 201 125 250 89 71 240 173 212 162 175 156 164 114 192 183 253 147 38 54 63 247 204 52 165 229 241 113 216 49 21 4 199 35 195 24 150 5 154 7 18 128 226 235 39 178 117 9 131 44 26 27 110 90 160 82 59 214 179 41 227 47 132 83 209 0 237 32 252 177 91 106 203 190 57 74 76 88 207 208 239 170 251 67 77 51 133 69 249 2 127 80 60 159 168 81 163 64 143 146 157 56 245 188 182 218 33 16 255 243 210 205 12 19 236 95 151 68 23 196 167 126 61 100 93 25 115 96 129 79 220 34 42 144 136 70 238 184 20 222 94 11 219 224 50 58 10 73 6 36 92 194 211 172 98 145 149 228 121 231 200 55 109 141 213 78 169 108 86 244 234 101 122 174 8 186 120 37 46 28 166 180 198 232 221 116 31 75 189 139 138 112 62 181 102 72 3 246 14 97 53 87 185 134 193 29 158 225 248 152 17 105 217 142 148 155 30 135 233 206 85 40 223 140 161 137 13 191 230 66 104 65 153 45 15 176 84 187 22]  syn_rom_auto_wl=off  syn_out_wl=8  syn_out_fl=0  syn_out_dt=unsigned  syn_out_sat=on  syn_out_rnd=on  syn_en_port=off  synBlockType=primitive  synLatency=1  synBlockId=62  syn_dual_port=on
  Sequence : shlslibv1/Sources/Sequence  syn_seq_vec=[0 1 0 2 0 1 0 1 0]  syn_seq_wl=8  syn_seq_fl=0  syn_seq_dt=unsigned  syn_rst_port=off  syn_en_port=off  syn_seq_st=-1  synBlockType=custom  synLatency=1
  Out1 : Outport
  wires:
  Extract1/1 -> Extract8/1, Extract6/1, Extract7/1, Extract5/1
  Extract2/1 -> Extract9/1, Extract12/1, Extract11/1, Extract10/1
  Extract3/1 -> Extract16/1, Extract14/1, Extract15/1, Extract13/1
  Extract4/1 -> Extract20/1, Extract18/1, Extract19/1, Extract17/1
  Extract5/1 -> Binary Logic16/2, ROM/1
  Extract6/1 -> Binary Logic17/2, ROM/2
  Extract7/1 -> Binary Logic18/2, ROM1/1
  Constant4/1 -> Mux/2
  Constant5/1 -> Mux/3
  Constant6/1 -> Mux/4
  Constant7/1 -> Mux/5
  Constant8/1 -> Mux/10
  Constant9/1 -> Mux/9
  Constant10/1 -> Mux/8
  Constant11/1 -> Mux/7
  Constant12/1 -> Mux/6
  Sequence/1 -> Mux/1
  ROM/1 -> Binary Logic/1
  Extract18/1 -> Binary Logic/2
  ROM/2 -> Binary Logic1/1
  Extract19/1 -> Binary Logic1/2
  ROM1/1 -> Binary Logic2/1
  Extract20/1 -> Binary Logic2/2
  ROM1/2 -> Binary Logic3/1
  Extract17/1 -> Binary Logic3/2
  Binary Logic2/1 -> Binary Logic7/1
  Mux/1 -> Binary Logic7/2
  Binary Logic/1 -> Binary Logic4/1
  Constant/1 -> Binary Logic4/2
  Constant1/1 -> Binary Logic5/2
  Binary Logic1/1 -> Binary Logic5/1
  Constant2/1 -> Binary Logic6/1
  Binary Logic3/1 -> Binary Logic6/2
  Binary Logic6/1 -> Concat2/3, Binary Logic11/1
  Extract16/1 -> Binary Logic11/2
  Binary Logic7/1 -> Concat2/4, Binary Logic8/1
  Extract13/1 -> Binary Logic8/2
  Extract14/1 -> Binary Logic9/2
  Binary Logic4/1 -> Concat2/1, Binary Logic9/1
  Binary Logic5/1 -> Concat2/2, Binary Logic10/1
  Extract15/1 -> Binary Logic10/2
  Extract9/1 -> Binary Logic12/2
  Binary Logic8/1 -> Concat/1, Binary Logic12/1
  Extract10/1 -> Binary Logic13/2
  Binary Logic9/1 -> Binary Logic13/1, Concat/2
  Extract11/1 -> Binary Logic14/2
  Binary Logic10/1 -> Binary Logic14/1, Concat/3
  Extract12/1 -> Binary Logic15/2
  Binary Logic11/1 -> Concat/4, Binary Logic15/1
  Binary Logic12/1 -> Binary Logic16/1, Concat1/1
  Binary Logic13/1 -> Concat1/2, Binary Logic17/1
  Binary Logic14/1 -> Concat1/3, Binary Logic18/1
  Binary Logic15/1 -> Binary Logic19/1, Concat1/4
  Extract8/1 -> Binary Logic19/2, ROM1/2
  Binary Logic16/1 -> Concat3/1
  Binary Logic17/1 -> Concat3/2
  Binary Logic19/1 -> Concat3/4
  Binary Logic18/1 -> Concat3/3
  Concat2/1 -> Concat4/1
  Concat/1 -> Concat4/2
  Concat1/1 -> Concat4/3
  Concat3/1 -> Concat4/4
  In1/1 -> Extract3/1, Extract4/1, Extract2/1, Extract1/1
  Concat4/1 -> Out1/1

== system unrolling_1/AES /Subsystem1/SB_rs_MIX_COLUMN ==
  In1 : Inport
  In2 : Inport  Port=2
  In3 : Inport  Port=3
  In4 : Inport  Port=4
  Concat{,1..4} (5 alike) : shlslibv1/Signal Operations/Concat  syn_in_nb=4  syn_out_f=Automatic  syn_out_wl=16  syn_out_fl=8  syn_out_dt=signed  syn_en_se=off  synBlockType=primitive  synLatency=0  synBlockId=8
  Extract{,4,8,12} (4 alike) : shlslibv1/Signal Operations/Extract  syn_extract_vec=[24:31]  synBlockType=primitive  synLatency=0  synBlockId=17
  Extract{1,5,9,13} (4 alike) : shlslibv1/Signal Operations/Extract  syn_extract_vec=[16:23]  synBlockType=primitive  synLatency=0  synBlockId=17
  Extract{2,6,10,14} (4 alike) : shlslibv1/Signal Operations/Extract  syn_extract_vec=[8:15]  synBlockType=primitive  synLatency=0  synBlockId=17
  Extract{3,7,11,15} (4 alike) : shlslibv1/Signal Operations/Extract  syn_extract_vec=[0:7]  synBlockType=primitive  synLatency=0  synBlockId=17
  ROM{,1..7} (8 alike) : shlslibv1/Memories/ROM  syn_rom_vec=[99 124 119 123 242 107 111 197 48 1 103 43 254 215 171 118 202 130 201 125 250 89 71 240 173 212 162 175 156 164 114 192 183 253 147 38 54 63 247 204 52 165 229 241 113 216 49 21 4 199 35 195 24 150 5 154 7 18 128 226 235 39 178 117 9 131 44 26 27 110 90 160 82 59 214 179 41 227 47 132 83 209 0 237 32 252 177 91 106 203 190 57 74 76 88 207 208 239 170 251 67 77 51 133 69 249 2 127 80 60 159 168 81 163 64 143 146 157 56 245 188 182 218 33 16 255 243 210 205 12 19 236 95 151 68 23 196 167 126 61 100 93 25 115 96 129 79 220 34 42 144 136 70 238 184 20 222 94 11 219 224 50 58 10 73 6 36 92 194 211 172 98 145 149 228 121 231 200 55 109 141 213 78 169 108 86 244 234 101 122 174 8 186 120 37 46 28 166 180 198 232 221 116 31 75 189 139 138 112 62 181 102 72 3 246 14 97 53 87 185 134 193 29 158 225 248 152 17 105 217 142 148 155 30 135 233 206 85 40 223 140 161 137 13 191 230 66 104 65 153 45 15 176 84 187 22]  syn_rom_auto_wl=off  syn_out_wl=8  syn_out_fl=0  syn_out_dt=unsigned  syn_out_sat=on  syn_out_rnd=on  syn_en_port=off  synBlockType=primitive  synLatency=1  synBlockId=62  syn_dual_port=on
  Subsystem : Subsystem
  Subsystem1 : Subsystem
  Subsystem2 : Subsystem
  Subsystem3 : Subsystem
  Out1 : Outport
  wires:
  Extract/1 -> ROM/1
  Extract1/1 -> ROM/2
  Extract2/1 -> ROM1/1
  Extract3/1 -> ROM1/2
  Extract4/1 -> ROM2/1
  Extract5/1 -> ROM2/2
  Extract6/1 -> ROM3/1
  Extract7/1 -> ROM3/2
  Extract8/1 -> ROM4/1
  Extract9/1 -> ROM4/2
  Extract10/1 -> ROM5/1
  Extract11/1 -> ROM5/2
  Extract12/1 -> ROM6/1
  Extract13/1 -> ROM6/2
  Extract14/1 -> ROM7/1
  Extract15/1 -> ROM7/2
  ROM1/2 -> Subsystem/1(In1)
  ROM7/1 -> Subsystem/2(In2)
  ROM4/2 -> Subsystem/3(In3)
  ROM2/1 -> Subsystem/4(In4)
  ROM3/2 -> Subsystem1/1(In1)
  ROM1/1 -> Subsystem1/2(In2)
  ROM6/2 -> Subsystem1/3(In3)
  ROM4/1 -> Subsystem1/4(In4)
  ROM5/2 -> Subsystem2/1(In1)
  ROM3/1 -> Subsystem2/2(In2)
  ROM/2 -> Subsystem2/3(In3)
  ROM6/1 -> Subsystem2/4(In4)
  ROM7/2 -> Subsystem3/1(In1)
  ROM5/1 -> Subsystem3/2(In2)
  ROM2/2 -> Subsystem3/3(In3)
  ROM/1 -> Subsystem3/4(In4)
  In1/1 -> Extract2/1, Extract3/1, Extract/1, Extract1/1
  In2/1 -> Extract6/1, Extract7/1, Extract4/1, Extract5/1
  In3/1 -> Extract10/1, Extract11/1, Extract9/1, Extract8/1
  In4/1 -> Extract12/1, Extract13/1, Extract15/1, Extract14/1
  Subsystem/1(Out1) -> Concat1/1
  Subsystem/2(Out2) -> Concat1/2
  Subsystem/3(Out3) -> Concat1/3
  Subsystem/4(Out4) -> Concat1/4
  Subsystem1/1(Out1) -> Concat2/1
  Subsystem1/2(Out2) -> Concat2/2
  Subsystem1/3(Out3) -> Concat2/3
  Subsystem1/4(Out4) -> Concat2/4
  Subsystem2/1(Out1) -> Concat3/1
  Subsystem2/2(Out2) -> Concat3/2
  Subsystem2/3(Out3) -> Concat3/3
  Subsystem2/4(Out4) -> Concat3/4
  Subsystem3/1(Out1) -> Concat4/1
  Subsystem3/2(Out2) -> Concat4/2
  Subsystem3/3(Out3) -> Concat4/3
  Subsystem3/4(Out4) -> Concat4/4
  Concat1/1 -> Concat/1
  Concat2/1 -> Concat/2
  Concat3/1 -> Concat/3
  Concat4/1 -> Concat/4
  Concat/1 -> Out1/1

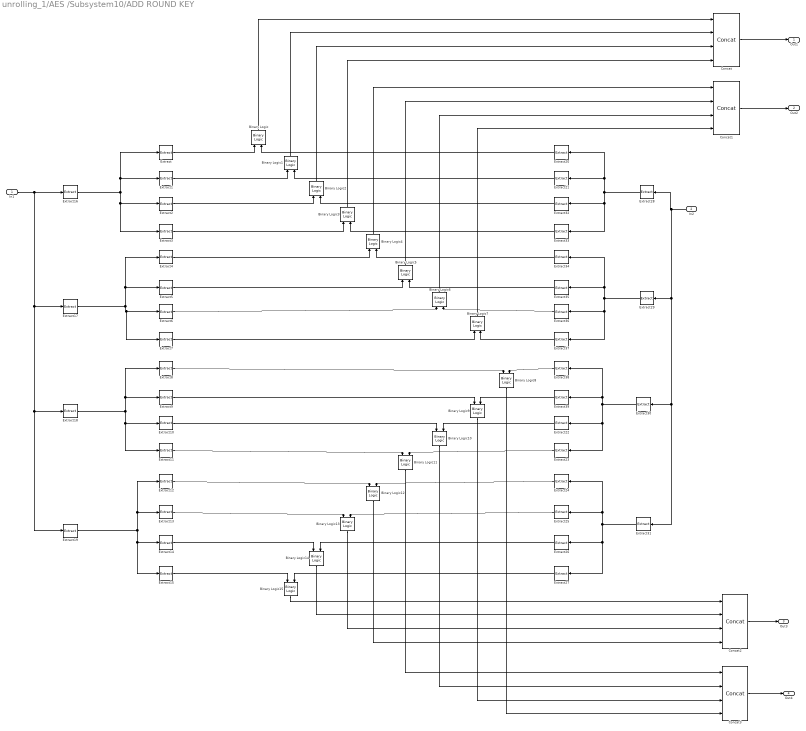
== system unrolling_1/AES /Subsystem10/ADD ROUND KEY ==
  In1 : Inport
  In2 : Inport  Port=2
  Binary Logic{,1..15} (16 alike) : shlslibv1/Math Functions/Binary Logic  syn_binlog_exp=a^b  synBlockType=primitive  synLatency=0  synBlockId=13
  Concat{,1..3} (4 alike) : shlslibv1/Signal Operations/Concat  syn_in_nb=4  syn_out_f=Automatic  syn_out_wl=16  syn_out_fl=8  syn_out_dt=signed  syn_en_se=off  synBlockType=primitive  synLatency=0  synBlockId=8
  Extract{,4,8,12,20,24,34,38} (8 alike) : shlslibv1/Signal Operations/Extract  syn_extract_vec=[24:31]  synBlockType=primitive  synLatency=0  synBlockId=17
  Extract{1,5,9,13,21,25,35,39} (8 alike) : shlslibv1/Signal Operations/Extract  syn_extract_vec=[16:23]  synBlockType=primitive  synLatency=0  synBlockId=17
  Extract{2,6,10,14,22,26,32,36} (8 alike) : shlslibv1/Signal Operations/Extract  syn_extract_vec=[8:15]  synBlockType=primitive  synLatency=0  synBlockId=17
  Extract{3,7,11,15,23,27,33,37} (8 alike) : shlslibv1/Signal Operations/Extract  syn_extract_vec=[0:7]  synBlockType=primitive  synLatency=0  synBlockId=17
  Extract16 : shlslibv1/Signal Operations/Extract  syn_extract_vec=[96:127]  synBlockType=primitive  synLatency=0  synBlockId=17
  Extract17 : shlslibv1/Signal Operations/Extract  syn_extract_vec=[64:95]  synBlockType=primitive  synLatency=0  synBlockId=17
  Extract18 : shlslibv1/Signal Operations/Extract  syn_extract_vec=[32:63]  synBlockType=primitive  synLatency=0  synBlockId=17
  Extract19 : shlslibv1/Signal Operations/Extract  syn_extract_vec=[0:31]  synBlockType=primitive  synLatency=0  synBlockId=17
  Extract28 : shlslibv1/Signal Operations/Extract  syn_extract_vec=[96:127]  synBlockType=primitive  synLatency=0  synBlockId=17
  Extract29 : shlslibv1/Signal Operations/Extract  syn_extract_vec=[64:95]  synBlockType=primitive  synLatency=0  synBlockId=17
  Extract30 : shlslibv1/Signal Operations/Extract  syn_extract_vec=[32:63]  synBlockType=primitive  synLatency=0  synBlockId=17
  Extract31 : shlslibv1/Signal Operations/Extract  syn_extract_vec=[0:31]  synBlockType=primitive  synLatency=0  synBlockId=17
  Out1 : Outport
  Out2 : Outport  Port=2
  Out3 : Outport  Port=3
  Out4 : Outport  Port=4
  wires:
  Extract16/1 -> Extract/1, Extract1/1, Extract2/1, Extract3/1
  Extract17/1 -> Extract6/1, Extract7/1, Extract4/1, Extract5/1
  Extract18/1 -> Extract9/1, Extract8/1, Extract10/1, Extract11/1
  Extract19/1 -> Extract12/1, Extract13/1, Extract15/1, Extract14/1
  In1/1 -> Extract19/1, Extract18/1, Extract17/1, Extract16/1
  In2/1 -> Extract31/1, Extract30/1, Extract29/1, Extract28/1
  Extract28/1 -> Extract21/1, Extract20/1, Extract33/1, Extract32/1
  Extract29/1 -> Extract35/1, Extract34/1, Extract36/1, Extract37/1
  Extract30/1 -> Extract23/1, Extract22/1, Extract38/1, Extract39/1
  Extract31/1 -> Extract24/1, Extract25/1, Extract27/1, Extract26/1
  Extract/1 -> Binary Logic/1
  Extract20/1 -> Binary Logic/2
  Extract1/1 -> Binary Logic1/1
  Extract21/1 -> Binary Logic1/2
  Extract2/1 -> Binary Logic2/1
  Extract32/1 -> Binary Logic2/2
  Extract3/1 -> Binary Logic3/1
  Extract33/1 -> Binary Logic3/2
  Extract4/1 -> Binary Logic4/1
  Extract34/1 -> Binary Logic4/2
  Extract5/1 -> Binary Logic5/1
  Extract35/1 -> Binary Logic5/2
  Extract6/1 -> Binary Logic6/1
  Extract36/1 -> Binary Logic6/2
  Extract7/1 -> Binary Logic7/1
  Extract37/1 -> Binary Logic7/2
  Extract8/1 -> Binary Logic8/1
  Extract38/1 -> Binary Logic8/2
  Extract9/1 -> Binary Logic9/1
  Extract39/1 -> Binary Logic9/2
  Extract22/1 -> Binary Logic10/2
  Extract10/1 -> Binary Logic10/1
  Extract23/1 -> Binary Logic11/2
  Extract11/1 -> Binary Logic11/1
  Extract12/1 -> Binary Logic12/1
  Extract24/1 -> Binary Logic12/2
  Extract13/1 -> Binary Logic13/1
  Extract25/1 -> Binary Logic13/2
  Extract14/1 -> Binary Logic14/1
  Extract26/1 -> Binary Logic14/2
  Extract15/1 -> Binary Logic15/1
  Extract27/1 -> Binary Logic15/2
  Binary Logic7/1 -> Concat1/4
  Binary Logic6/1 -> Concat1/3
  Binary Logic5/1 -> Concat1/2
  Binary Logic4/1 -> Concat1/1
  Binary Logic3/1 -> Concat/4
  Binary Logic2/1 -> Concat/3
  Binary Logic1/1 -> Concat/2
  Binary Logic/1 -> Concat/1
  Binary Logic15/1 -> Concat2/1
  Binary Logic14/1 -> Concat2/2
  Binary Logic13/1 -> Concat2/3
  Binary Logic12/1 -> Concat2/4
  Binary Logic11/1 -> Concat3/1
  Binary Logic10/1 -> Concat3/2
  Binary Logic9/1 -> Concat3/3
  Binary Logic8/1 -> Concat3/4
  Concat/1 -> Out1/1
  Concat1/1 -> Out2/1
  Concat2/1 -> Out3/1
  Concat3/1 -> Out4/1
